simulink library "calcTangentialCoord_ul"  (R2020a)
settings: Solver=VariableStepAuto  StartTime=0.0  StopTime=10.0  RelTol=1e-3
settings Model: Creator=Ayaz  LastModifiedBy=Ayaz

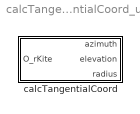
== system calcTangentialCoord_ul ==
  calcTangentialCoord : Subsystem

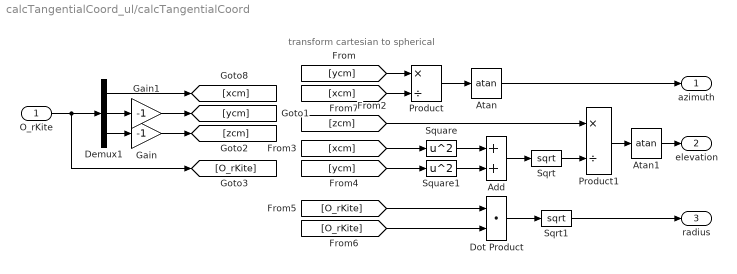
== system calcTangentialCoord_ul/calcTangentialCoord ==
  note: transform cartesian to spherical
  O_rKite : Inport
  Add : Sum
  Atan : Trigonometry  Operator=atan
  Atan1 : Trigonometry  Operator=atan
  Demux1 : Demux  Outputs=3
  Dot Product : DotProduct  InputSameDT=on  OutDataTypeStr=Inherit: Inherit via internal rule
  Gain : Gain  Gain=-1
  Gain1 : Gain  Gain=-1
  Product : Product  Inputs=*/
  Product1 : Product  Inputs=*/
  Sqrt : Sqrt  SaturateOnIntegerOverflow=on
  Sqrt1 : Sqrt  SaturateOnIntegerOverflow=on
  Square : Math  Operator=square  SaturateOnIntegerOverflow=on
  Square1 : Math  Operator=square  SaturateOnIntegerOverflow=on
  azimuth : Outport
  elevation : Outport  Port=2
  radius : Outport  Port=3
  wires:
  O_rKite/1 -> [O_rKite], Demux1/1
  Demux1/1 -> [xcm]
  Demux1/2 -> Gain1/1
  Demux1/3 -> Gain/1
  [ycm] -> Product/1
  [xcm] -> Product/2
  Product/1 -> Atan/1
  Atan/1 -> azimuth/1
  [xcm] -> Square/1
  [ycm] -> Square1/1
  Square1/1 -> Add/2
  Square/1 -> Add/1
  Add/1 -> Sqrt/1
  Sqrt/1 -> Product1/2
  [zcm] -> Product1/1
  Product1/1 -> Atan1/1
  [O_rKite] -> Dot Product/1
  [O_rKite] -> Dot Product/2
  Dot Product/1 -> Sqrt1/1
  Sqrt1/1 -> radius/1
  Gain/1 -> [zcm]
  Atan1/1 -> elevation/1
  Gain1/1 -> [ycm]
